simulink model "Project_MATLAB_diagram"  (R2016a)
settings: Solver=FixedStepDiscrete  StartTime=0.0  StopTime=inf  FixedStep=0.1  RelTol=1e-3
libraries: arduinolib x8
settings Model: SimulationMode=external  ExtModeTrigDuration=2  Creator=Mostafa  LastModifiedBy=Mostafa
settings SolverCC: AutoInsertRateTranBlk=on
settings DataIOCC: LimitDataPoints=on
settings OptimizationCC: OptimizeModelRefInitCode=on  LifeSpan=Inf  MaxStackSize=64
settings DebuggingCC: AllowSymbolicDim=off
settings HardwareCC: ProdBitPerInt=16  ProdBitPerPointer=16  ProdLargestAtomicFloat=None  ProdWordSize=8  ProdHWDeviceType=Atmel->AVR
settings RTWCC: SystemTargetFile=ert.tlc  HardwareBoard=Arduino Uno  TemplateMakefile=ert_default_tmf  GenerateReport=on  Toolchain=Arduino AVR v1.6.1  BuildConfiguration=Faster Runs  IncludeHyperlinkInReport=on  LaunchReport=on  GenerateTraceInfo=on  GenerateTraceReport=on  GenerateTraceReportSl=on  GenerateTraceReportSf=on  GenerateTraceReportEml=on
settings CodeAppCC: ForceParamTrailComments=on  IgnoreCustomStorageClasses=off  OperatorAnnotations=on  SimulinkDataObjDesc=on  SFDataObjDesc=on  MATLABFcnDesc=on  InsertBlockDesc=on  MATLABSourceComments=on
settings ERTTargetCC: SupportContinuousTime=on  SupportVariableSizeSignals=on
settings ConfigComp: CovModelRefEnable=Off  CovSFcnEnable=off

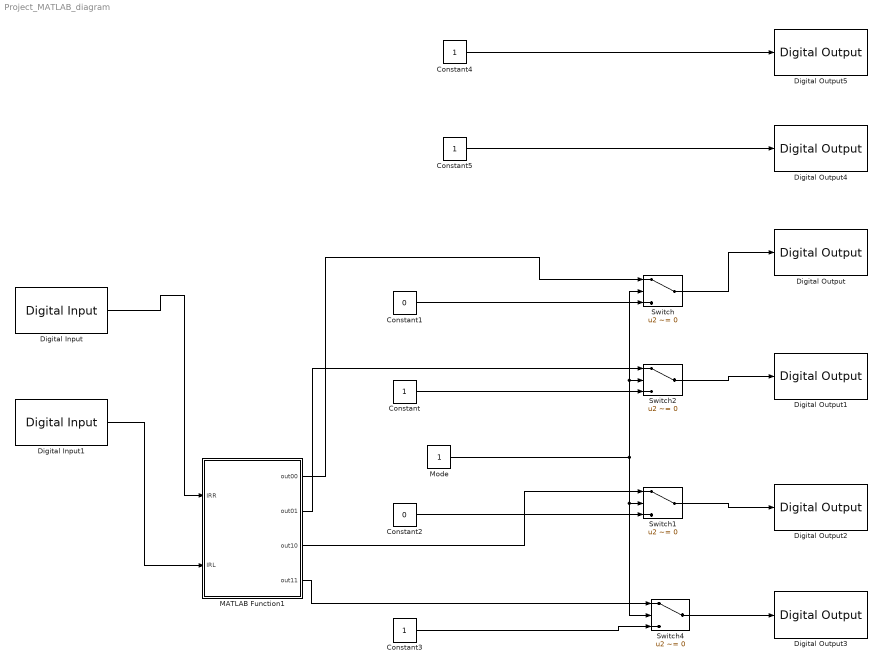
== system Project_MATLAB_diagram ==
  Constant{,3..5} (4 alike) : Constant
  Constant1 : Constant  Value=0
  Constant2 : Constant  Value=0
  Digital Input : arduinolib/Digital Input  pinNumber=3  sampleTime=1  blockPlatform=arduino
  Digital Input1 : arduinolib/Digital Input  pinNumber=5  sampleTime=1  blockPlatform=arduino
  Digital Output : arduinolib/Digital Output  pinNumber=8  blockPlatform=arduino
  Digital Output1 : arduinolib/Digital Output  pinNumber=9  blockPlatform=arduino
  Digital Output2 : arduinolib/Digital Output  pinNumber=12  blockPlatform=arduino
  Digital Output3 : arduinolib/Digital Output  pinNumber=13  blockPlatform=arduino
  Digital Output4 : arduinolib/Digital Output  pinNumber=11  blockPlatform=arduino
  Digital Output5 : arduinolib/Digital Output  pinNumber=10  blockPlatform=arduino
  MATLAB Function1 : MATLAB Function  TreatAsAtomicUnit=on
  Mode : Constant
  Switch{,1..2,4} (4 alike) : Switch  Criteria=u2 ~= 0
  wires:
  Digital Input1/1 -> MATLAB Function1/2(IRL)
  Digital Input/1 -> MATLAB Function1/1(IRR)
  MATLAB Function1/1(out00) -> Switch/1
  Constant1/1 -> Switch/3
  Constant/1 -> Switch2/3
  MATLAB Function1/2(out01) -> Switch2/1
  MATLAB Function1/3(out10) -> Switch1/1
  MATLAB Function1/4(out11) -> Switch4/1
  Constant2/1 -> Switch1/3
  Constant3/1 -> Switch4/3
  Mode/1 -> Switch/2, Switch2/2, Switch4/2, Switch1/2
  Switch/1 -> Digital Output/1
  Switch2/1 -> Digital Output1/1
  Switch1/1 -> Digital Output2/1
  Switch4/1 -> Digital Output3/1
  Constant4/1 -> Digital Output5/1
  Constant5/1 -> Digital Output4/1

== matlab function Project_MATLAB_diagram/MATLAB Function1 ==
  data: IRR input; out00 output; IRL input; out01 output; out10 output; out11 output
function [out00,out01,out10,out11] = fcn(IRR,IRL)
%#codegen
if(IRR == 0 & IRL == 0)
    out00 = 0;
    out01 = 1;
    out10 = 0;
    out11 = 1;
elseif(IRR == 1 & IRL == 0)
    out00 = 0;
    out01 = 0;
    out10 = 0;
    out11 = 1;
elseif(IRR == 0 & IRL == 1)
    out00 = 0;
    out01 = 1;
    out10 = 0;
    out11 = 0;
elseif(IRR == 1 & IRL == 1)
    out00 = 0;
    out01 = 0;
    out10 = 0;
    out11 = 0;
else
    out00 = 1;
    out01 = 0;
    out10 = 1;
    out11 = 0;
end
